simulink model "Sim_Main"  (R2020b)
settings: Solver=VariableStepAuto  StartTime=0.0  StopTime=150.0  RelTol=1e-3
values from neighbouring files (symbols this model uses):
  A_ob = [(A_oc + (Lx * C_oc))    Lx ... (first row only)    [observer_calc.m]
  B_ob = B_oc    [observer_calc.m]
  C_ob = [Lx ... (first row only)    [observer_calc.m]
undefined symbols (not defined in the file or in its folder): A_ct, B_ct, C_ct, D_ct
settings Model: Creator=andrewralea  LastModifiedBy=andrewralea

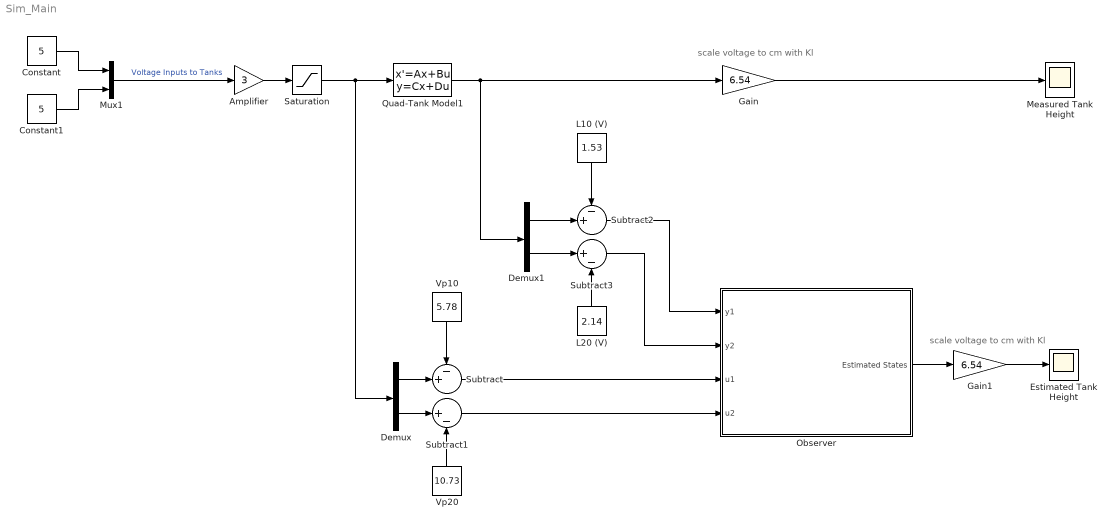
== system Sim_Main ==
  note: scale voltage to cm with Kl
  note: scale voltage to cm with Kl
  Amplifier : Gain  Gain=3
  Constant : Constant  Value=5
  Constant1 : Constant  Value=5
  Demux : Demux  Outputs=2
  Demux1 : Demux  Outputs=2
  Estimated Tank Height : Scope
  Gain : Gain  Gain=6.54
  Gain1 : Gain  Gain=6.54
  L10 (V) : Constant  Value=1.53
  L20 (V) : Constant  Value=2.14
  Measured Tank Height : Scope
  Mux1 : Mux  Inputs=2
  Observer : Subsystem
  Quad-Tank Model1 : StateSpace  A=A_ct  B=B_ct  C=C_ct  D=D_ct  InitialCondition=[]
  Saturation : Saturate  UpperLimit=22  LowerLimit=0
  Subtract : Sum  Inputs=-+|
  Subtract1 : Sum  Inputs=|+-
  Subtract2 : Sum  Inputs=-+|
  Subtract3 : Sum  Inputs=|+-
  Vp10 : Constant  Value=5.78
  Vp20 : Constant  Value=10.73
  wires:
  Constant/1 -> Mux1/1
  Constant1/1 -> Mux1/2
  Mux1/1 -> Amplifier/1  "Voltage Inputs to Tanks"
  Quad-Tank Model1/1 -> Demux1/1, Gain/1
  Gain/1 -> Measured Tank Height/1
  Amplifier/1 -> Saturation/1
  Saturation/1 -> Demux/1, Quad-Tank Model1/1
  Vp20/1 -> Subtract1/2
  Demux/1 -> Subtract/2
  Vp10/1 -> Subtract/1
  Demux/2 -> Subtract1/1
  Subtract1/1 -> Observer/4(u2)
  Subtract/1 -> Observer/3(u1)
  Observer/1(Estimated States) -> Gain1/1
  Gain1/1 -> Estimated Tank Height/1
  L10 (V)/1 -> Subtract2/1
  L20 (V)/1 -> Subtract3/2
  Demux1/1 -> Subtract2/2
  Demux1/2 -> Subtract3/1
  Subtract3/1 -> Observer/2(y2)
  Subtract2/1 -> Observer/1(y1)

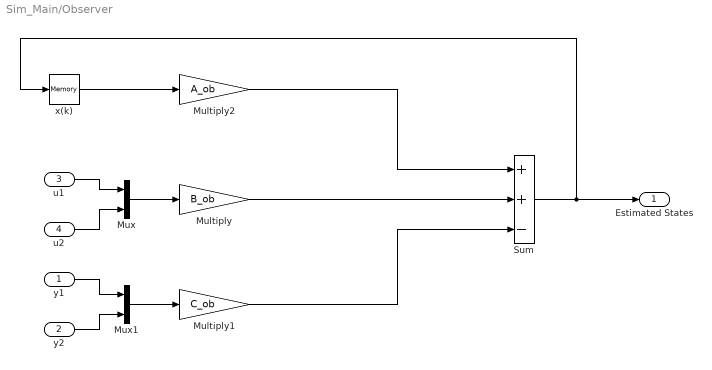
== system Sim_Main/Observer ==
  y1 : Inport
  y2 : Inport  Port=2
  u1 : Inport  Port=3
  u2 : Inport  Port=4
  Multiply : Gain  Gain=B_ob
  Multiply1 : Gain  Gain=C_ob
  Multiply2 : Gain  Gain=A_ob
  Mux : Mux  Inputs=2
  Mux1 : Mux  Inputs=2
  Sum : Sum  Inputs=++-
  x(k) : Memory  InitialCondition=[0; 0; 0; 0; 0; 0; 0; 0; 0; 0]
  Estimated States : Outport
  wires:
  Sum/1 -> x(k)/1, Estimated States/1
  Multiply/1 -> Sum/2
  y1/1 -> Mux1/1
  y2/1 -> Mux1/2
  Mux1/1 -> Multiply1/1
  Multiply1/1 -> Sum/3
  Multiply2/1 -> Sum/1
  Mux/1 -> Multiply/1
  u1/1 -> Mux/1
  u2/1 -> Mux/2
  x(k)/1 -> Multiply2/1
